simulink library "GUARD_Toolbox"  (R2016a)
settings: Solver=ode45  StartTime=0.0  StopTime=10.0  RelTol=1e-3
undefined symbols (not defined in the file): beta_s, DiscIntNeverNeededParam, k_s, Ts, UW
libraries: vrlib x7, GUARD_Toolbox x3, instrumentlib x1
settings Model: Creator=Marlo  LastModifiedBy=marlo
settings DataIOCC: LimitDataPoints=on
settings DebuggingCC: AllowSymbolicDim=off

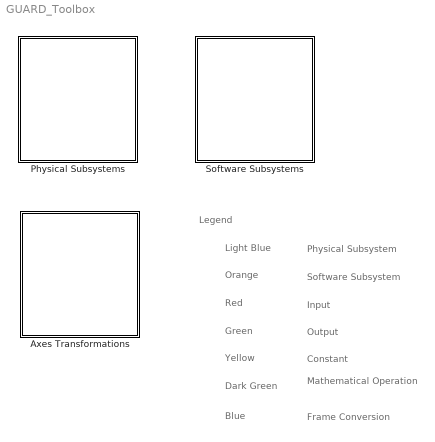
== system GUARD_Toolbox ==
  note: Legend
  note: Physical Subsystem
  note: Light Blue
  note: Red
  note: Input
  note: Green
  note: Output
  note: Yellow
  note: Constant
  note: Dark Green
  note: Mathematical
      | Operation
  note: Software Subsystem
  note: Orange
  note: Blue
  note: Frame Conversion
  Axes Transformations : Subsystem
      mask Display: image(fullfile('Icons','coord_sys.png'));
  Physical Subsystems : Subsystem
      mask Display: image(fullfile('Icons','SS_ISS_low.jpg'));
  Software Subsystems : Subsystem
      mask Display: image(fullfile('Icons','GPAD.png'));

== system GUARD_Toolbox/Axes Transformations ==
  Body to ECI : MATLAB Function  TreatAsAtomicUnit=on  mask(Body to ECI){}
      mask help: Converts a vector in the body frame to an equivalent one in the ECI frame.
  ECI to Body : MATLAB Function  TreatAsAtomicUnit=on  mask(ECI to body){}
      mask help: Converts a vector in the ECI frame to an equivalent one in the body frame.
  From ECEF to ECI : MATLAB Function  TreatAsAtomicUnit=on  mask(ECEF to ECI){}
      mask help: Convert Earth Centered Earth Fixed (ECEF) coordinates to Earth Centered Inertial (ECI) coordinates.
  From ECEF to LLA : MATLAB Function  TreatAsAtomicUnit=on  mask(ECEF to LLA){}
      mask help: Convert Earth Centered Earth Fixed (ECEF) coordinates to Latitude, Longitude, Altitude (LLA) geodetic coordinates.
  From ECI to ECEF : MATLAB Function  TreatAsAtomicUnit=on  mask(ECI to ECEF){}
      mask help: Convert Earth Centered Inertial (ECI) coordinates to Earth Centered Earth Fixed (ECEF) coordinates.
  From ECI to LLA : MATLAB Function  TreatAsAtomicUnit=on  mask(ECI to LLA){}
      mask help: Convert Earth Centered Inertial (ECI) coordinates to Latitude, Longitude, Altitude (LLA) geodetic coordinates.
  From LLA to ECEF : MATLAB Function  TreatAsAtomicUnit=on  mask(LLA to ECEF){}
      mask help: Convert Latitude, Longitude, Altitude (LLA) geodetic coordinates to Earth Centered Earth Fixed (ECEF) coordinates.
  From LVLH to ECI : MATLAB Function  TreatAsAtomicUnit=on  mask(LVLH to ECI){}
      mask help: Convert a vector from the Local Horizontal Local Vertical frame to the Earth Centered Inertial frame.

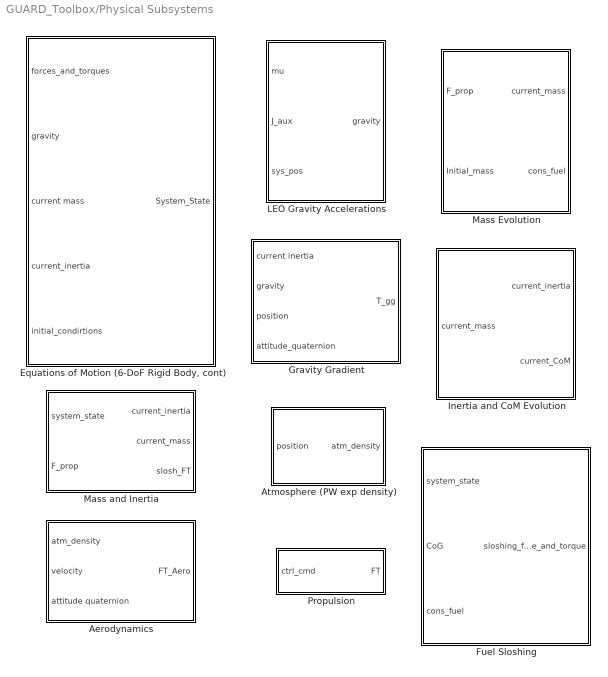
== system GUARD_Toolbox/Physical Subsystems ==
  Aerodynamics : Subsystem  mask(Aerodynamics Model){}
      mask help: Forces and torques enforced on the satellite due to the aerodynamic drag.
  Atmosphere (PW exp density) : Subsystem  mask(Piecewise Atmospheric Model){}
      mask help: U.S. Standard Atmosphere 1976 for 0 [Km], CIRA-72 for 25-500 [Km] and CIRA-72 with exospheric temperature Tinf = 1000 [K] for 500-1000 [Km].
  "Equations of Motion (6-DoF Rigid Body, cont)" : Subsystem  mask(Equatons of Motion){}
      mask help: Non-linear translational and rotational Equations of Motion for a rigid body with six degrees of freedom.
  Fuel Sloshing : Subsystem  mask(Fuel Sloshing){}
      mask help: Compute the disturbance forces and the torques generated by fuel sloshing via a mass-spring-dampener model.
  Gravity Gradient : Subsystem  mask(Gravity Gradient Torque){}
      mask help:
      | Compute the torques acting on the satellite's body due to the gravity gradient. The planet is assumed to be a perfect sphere with radially
      | symmetric mass distribution.
  Inertia and CoM Evolution : Subsystem  mask(Inertia and Center of Mass Evolution){}
      mask help: Interpolated lookup tables to compute the actual inertia matrix and center of mass.
  LEO Gravity Accelerations : MATLAB Function  TreatAsAtomicUnit=on  mask(LEO Gravity Model){}
      mask help: Compute the gravity acceleration vector for a small body in Low Earth Orbit (LEO) taking in account for J2 and J3 zonal harmonics perturbations due to the oblateness of the planet.
  Mass Evolution : Subsystem  mask(Mass Evolution){}
      mask help: Utilizes the forces generated by the propulsion system and the initial mass of the vehicle to compute the actual mass of the satellite and the consumed fuel.
  Mass and Inertia : Subsystem  mask(Preset Mass and Inertia Subsystem){}
      mask help: Mass and Inertia evolution using "Mass Evolution", "Inertia and CoM", and "Fuel Sloshing" blocks.
  Propulsion : Subsystem  mask(Propulson System){}
      mask help: Satellite's propulsion system.

== system GUARD_Toolbox/Software Subsystems ==
  Control Allocation : Subsystem  mask(Controll Allocator){}
      mask help: Allocate actuators.
  GNC : Subsystem  mask(GNC Subsystem){}
      mask help: Guidance Navigation and Control Architecture.
  State Estimation : Subsystem  mask(State Estimation){}
      mask help: Fuse sensors data to estimate the current system's state.
  UE4 OSC_UDP Interface : Subsystem  mask(UE4 OSC_UDP Interface){}
      mask help: Send data to the Unreal Engine 4 using the OSC protocol via UDP network.

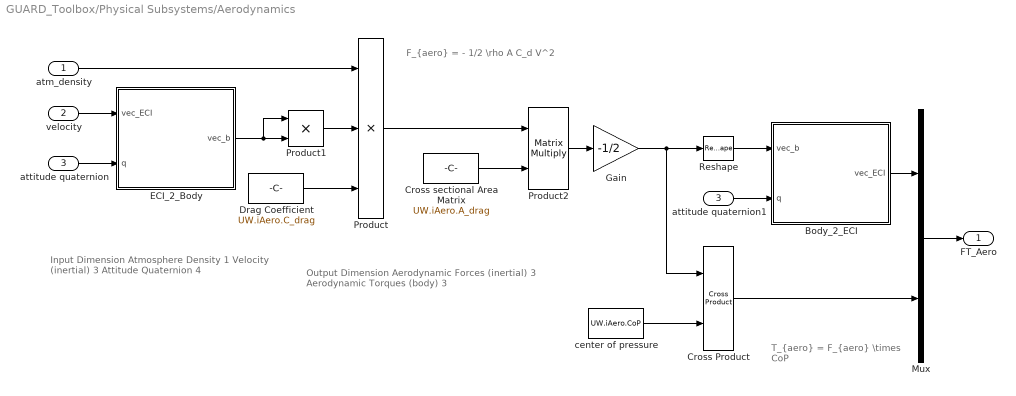
== system GUARD_Toolbox/Physical Subsystems/Aerodynamics ==
  note: F_{aero} = - 1/2 \rho A C_d V^2
  note: Input
      | Dimension
      |
      | Atmosphere Density
      | 1
      |
      | Velocity (inertial)
      | 3
      |
      | Attitude Quaternion
      | 4
  note: Output
      | Dimension
      |
      | Aerodynamic Forces (inertial)
      | 3
      |
      | Aerodynamic Torques (body)
      | 3
  note: T_{aero} = F_{aero} \times CoP
  atm_density : Inport
  velocity : Inport  Port=2
  attitude quaternion : Inport  Port=3
  Body_2_ECI : MATLAB Function  TreatAsAtomicUnit=on
  Cross Product : vrlib/Utilities/Cross Product
  Cross sectional Area Matrix : Constant  Value=UW.iAero.A_drag
  Drag Coefficient : Constant  Value=UW.iAero.C_drag
  ECI_2_Body : MATLAB Function  TreatAsAtomicUnit=on
  Gain : Gain  Gain=-1/2
  Mux : Mux  Inputs=[3 3]
  Product : Product  Inputs=***  SaturateOnIntegerOverflow=on  RndMeth=Zero  InputSameDT=on  OutDataTypeStr=Inherit: Same as first input
  Product1 : Product  Inputs=**  SaturateOnIntegerOverflow=on  RndMeth=Zero  InputSameDT=on  OutDataTypeStr=Inherit: Same as first input
  Product2 : Product  Inputs=**  Multiplication=Matrix(*)  SaturateOnIntegerOverflow=on  RndMeth=Zero  InputSameDT=on  OutDataTypeStr=Inherit: Same as first input
  Reshape : Reshape  OutputDimensionality=Column vector (2-D)
  attitude quaternion1 : InportShadow  Port=3
  center of pressure : Constant  Value=UW.iAero.CoP
  FT_Aero : Outport
  wires:
  Drag Coefficient/1 -> Product/3
  atm_density/1 -> Product/1
  Product1/1 -> Product/2
  Product/1 -> Product2/1
  Cross sectional Area Matrix/1 -> Product2/2
  Gain/1 -> Reshape/1, Cross Product/1
  Product2/1 -> Gain/1
  Cross Product/1 -> Mux/2
  velocity/1 -> ECI_2_Body/1(vec_ECI)
  attitude quaternion/1 -> ECI_2_Body/2(q)
  ECI_2_Body/1(vec_b) -> Product1/2, Product1/1
  center of pressure/1 -> Cross Product/2
  attitude quaternion1/1 -> Body_2_ECI/2(q)
  Body_2_ECI/1(vec_ECI) -> Mux/1
  Mux/1 -> FT_Aero/1
  Reshape/1 -> Body_2_ECI/1(vec_b)

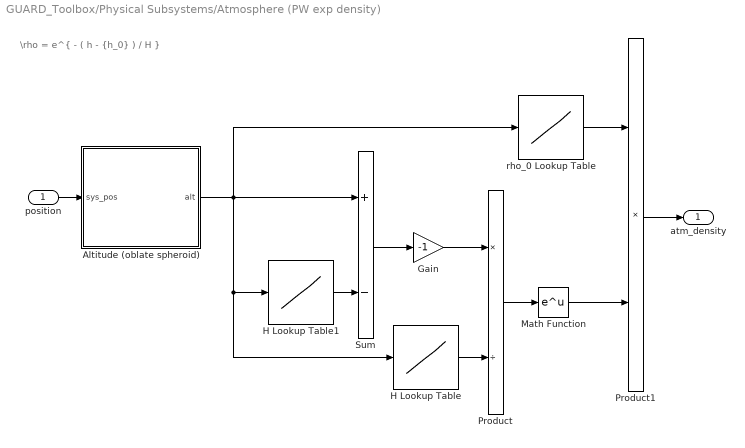
== system GUARD_Toolbox/Physical Subsystems/Atmosphere (PW exp density) ==
  note: \rho = e^{ - ( h - {h_0} ) / H }
  position : Inport
  Altitude (oblate spheroid) : MATLAB Function  TreatAsAtomicUnit=on
  Gain : Gain  Gain=-1
  H Lookup Table : Lookup_n-D  NumberOfTableDimensions=1  BreakpointsForDimension1=UW.iPWatm.h_idx  Table=UW.iPWatm.H  InternalRulePriority=Speed  RndMeth=Simplest  InputSameDT=on
  H Lookup Table1 : Lookup_n-D  NumberOfTableDimensions=1  BreakpointsForDimension1=UW.iPWatm.h_idx  Table=UW.iPWatm.h_idx  InternalRulePriority=Speed  RndMeth=Simplest  InputSameDT=on
  Math Function : Math  SaturateOnIntegerOverflow=on
  Product : Product  Inputs=*/  SaturateOnIntegerOverflow=on  RndMeth=Zero  InputSameDT=on  OutDataTypeStr=Inherit: Same as first input
  Product1 : Product  Inputs=**  SaturateOnIntegerOverflow=on  RndMeth=Zero  InputSameDT=on  OutDataTypeStr=Inherit: Same as first input
  Sum : Sum  Inputs=+-
  rho_0 Lookup Table : Lookup_n-D  NumberOfTableDimensions=1  BreakpointsForDimension1=UW.iPWatm.h_idx  Table=UW.iPWatm.rho_0  InternalRulePriority=Speed  RndMeth=Simplest  InputSameDT=on
  atm_density : Outport
  wires:
  Product1/1 -> atm_density/1
  position/1 -> Altitude (oblate spheroid)/1(sys_pos)
  Altitude (oblate spheroid)/1(alt) -> Sum/1, rho_0 Lookup Table/1, H Lookup Table/1, H Lookup Table1/1
  Sum/1 -> Gain/1
  Gain/1 -> Product/1
  H Lookup Table/1 -> Product/2
  Product/1 -> Math Function/1
  Math Function/1 -> Product1/2
  rho_0 Lookup Table/1 -> Product1/1
  H Lookup Table1/1 -> Sum/2

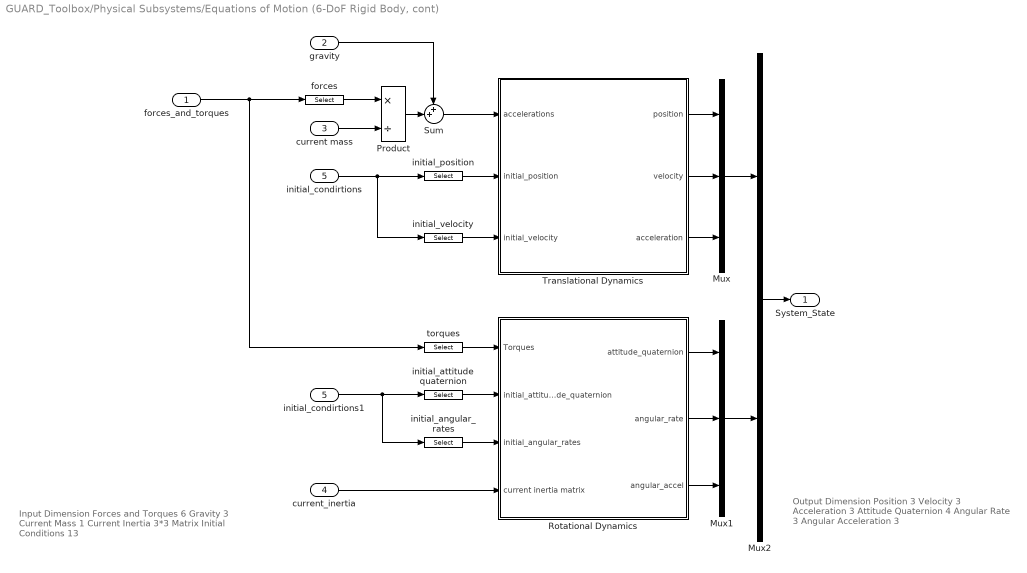
== system GUARD_Toolbox/Physical Subsystems/Equations of Motion (6-DoF Rigid Body, cont) ==
  note: Output
      | Dimension
      |
      | Position
      | 3
      |
      | Velocity
      | 3
      |
      | Acceleration
      | 3
      |
      | Attitude Quaternion
      | 4
      |
      | Angular Rate
      | 3
      |
      | Angular Acceleration
      | 3
  note: Input
      | Dimension
      |
      | Forces and Torques
      | 6
      |
      | Gravity
      | 3
      |
      | Current Mass
      | 1
      |
      | Current Inertia
      | 3*3 Matrix
      |
      | Initial Conditions
      | 13
  forces_and_torques : Inport
  gravity : Inport  Port=2
  current mass : Inport  Port=3  PortDimensions=1
  current_inertia : Inport  Port=4
  initial_condirtions : Inport  Port=5
  Mux : Mux  Inputs=[3 3 3]
  Mux1 : Mux  Inputs=[4 3 3]
  Mux2 : Mux  Inputs=[9 10]
  Product : Product  Inputs=*/  SaturateOnIntegerOverflow=on  RndMeth=Zero  InputSameDT=on  OutDataTypeStr=Inherit: Same as first input
  Rotational Dynamics : Subsystem
  Sum : Sum  Inputs=++|
  Translational Dynamics : Subsystem
  forces : Selector  InputPortWidth=6  IndexOptions=Index vector (dialog)  Indices=[1 2 3]  OutputSizes=1
  initial_angular_rates : Selector  InputPortWidth=13  IndexOptions=Index vector (dialog)  Indices=[11 12 13]  OutputSizes=1
  initial_attitude quaternion : Selector  InputPortWidth=13  IndexOptions=Index vector (dialog)  Indices=[7 8 9 10]  OutputSizes=1
  initial_condirtions1 : InportShadow  Port=5
  initial_position : Selector  InputPortWidth=13  IndexOptions=Index vector (dialog)  Indices=[1 2 3]  OutputSizes=1
  initial_velocity : Selector  InputPortWidth=13  IndexOptions=Index vector (dialog)  Indices=[4 5 6]  OutputSizes=1
  torques : Selector  InputPortWidth=6  IndexOptions=Index vector (dialog)  Indices=[4 5 6]  OutputSizes=1
  System_State : Outport
  wires:
  Mux1/1 -> Mux2/2
  Mux/1 -> Mux2/1
  Rotational Dynamics/1(attitude_quaternion) -> Mux1/1
  Rotational Dynamics/2(angular_rate) -> Mux1/2
  Rotational Dynamics/3(angular_accel) -> Mux1/3
  Translational Dynamics/1(position) -> Mux/1
  Translational Dynamics/2(velocity) -> Mux/2
  Translational Dynamics/3(acceleration) -> Mux/3
  Mux2/1 -> System_State/1
  initial_condirtions1/1 -> initial_attitude quaternion/1, initial_angular_rates/1
  initial_condirtions/1 -> initial_position/1, initial_velocity/1
  initial_attitude quaternion/1 -> Rotational Dynamics/2(initial_attitude_quaternion)
  initial_angular_rates/1 -> Rotational Dynamics/3(initial_angular_rates)
  initial_velocity/1 -> Translational Dynamics/3(initial_velocity)
  initial_position/1 -> Translational Dynamics/2(initial_position)
  current_inertia/1 -> Rotational Dynamics/4(current inertia matrix)
  torques/1 -> Rotational Dynamics/1(Torques)
  forces_and_torques/1 -> torques/1, forces/1
  gravity/1 -> Sum/1
  Sum/1 -> Translational Dynamics/1(accelerations)
  forces/1 -> Product/1
  current mass/1 -> Product/2
  Product/1 -> Sum/2

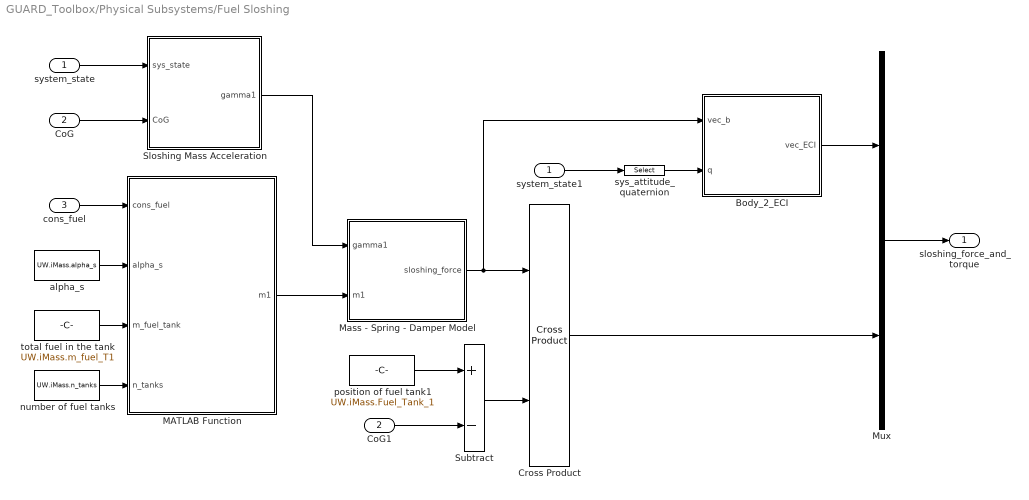
== system GUARD_Toolbox/Physical Subsystems/Fuel Sloshing ==
  system_state : Inport
  CoG : Inport  Port=2
  cons_fuel : Inport  Port=3
  Body_2_ECI : MATLAB Function  TreatAsAtomicUnit=on
  CoG1 : InportShadow  Port=2
  Cross Product : vrlib/Utilities/Cross Product
  MATLAB Function : MATLAB Function  TreatAsAtomicUnit=on
  Mass - Spring - Damper Model : Subsystem
  Mux : Mux  Inputs=[3 3]
  Sloshing Mass Acceleration : Subsystem
  Subtract : Sum  Inputs=+-
  alpha_s : Constant  Value=UW.iMass.alpha_s
  number of fuel tanks : Constant  Value=UW.iMass.n_tanks
  position of fuel tank1 : Constant  Value=UW.iMass.Fuel_Tank_1
  sys_attitude_quaternion : Selector  InputPortWidth=19  IndexOptions=Index vector (dialog)  Indices=[10 11 12 13]  OutputSizes=1
  system_state1 : InportShadow
  total fuel in the tank : Constant  Value=UW.iMass.m_fuel_T1
  sloshing_force_and_torque : Outport
  wires:
  system_state1/1 -> sys_attitude_quaternion/1
  sys_attitude_quaternion/1 -> Body_2_ECI/2(q)
  Sloshing Mass Acceleration/1(gamma1) -> Mass - Spring - Damper Model/1(gamma1)
  CoG1/1 -> Subtract/2
  position of fuel tank1/1 -> Subtract/1
  system_state/1 -> Sloshing Mass Acceleration/1(sys_state)
  CoG/1 -> Sloshing Mass Acceleration/2(CoG)
  Mux/1 -> sloshing_force_and_torque/1
  Body_2_ECI/1(vec_ECI) -> Mux/1
  Cross Product/1 -> Mux/2
  Subtract/1 -> Cross Product/2
  Mass - Spring - Damper Model/1(sloshing_force) -> Body_2_ECI/1(vec_b), Cross Product/1
  number of fuel tanks/1 -> MATLAB Function/4(n_tanks)
  cons_fuel/1 -> MATLAB Function/1(cons_fuel)
  MATLAB Function/1(m1) -> Mass - Spring - Damper Model/2(m1)
  total fuel in the tank/1 -> MATLAB Function/3(m_fuel_tank)
  alpha_s/1 -> MATLAB Function/2(alpha_s)

== system GUARD_Toolbox/Physical Subsystems/Gravity Gradient ==
  note: T_{gg} = 3 \mu / r^3 \bf{o_3} \times I o_3
  note: Output
      | Dimension
      |
      | Gravity Gradient Torque (body)
      | 3
  note: Input
      | Dimension
      |
      | Current Inertia
      | 3*3
      |
      | Position (inertial)
      | 3
      |
      | Attitude Quaternion
      | 4
  current inertia : Inport
  gravity : Inport  Port=2
  position : Inport  Port=3
  attitude_quaternion : Inport  Port=4
  ECI to Body : MATLAB Function  TreatAsAtomicUnit=on  mask(ECI to body){}
      mask help: Converts a vector in the ECI frame to an equivalent one in the body frame.
  Gravity Gradient Torque : MATLAB Function  TreatAsAtomicUnit=on
  gravitaitonal parameter : Constant  Value=UW.iPlanet.mu
  T_gg : Outport
  wires:
  current inertia/1 -> Gravity Gradient Torque/4(current_inertia)
  Gravity Gradient Torque/1(ggt) -> T_gg/1
  gravity/1 -> ECI to Body/1(vec_ECI)
  attitude_quaternion/1 -> ECI to Body/2(q)
  ECI to Body/1(vec_b) -> Gravity Gradient Torque/1(gravity_body)
  position/1 -> Gravity Gradient Torque/2(sys_pos)
  gravitaitonal parameter/1 -> Gravity Gradient Torque/3(mu)

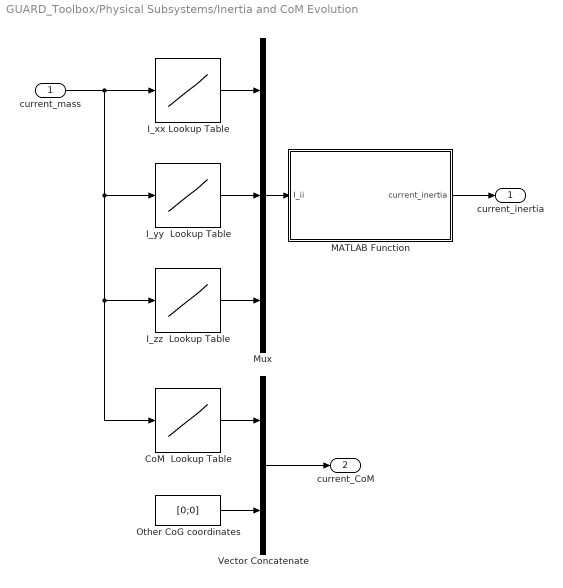
== system GUARD_Toolbox/Physical Subsystems/Inertia and CoM Evolution ==
  current_mass : Inport
  CoM  Lookup Table : Lookup_n-D  NumberOfTableDimensions=1  BreakpointsForDimension1=UW.iMass.m_idx  Table=UW.iMass.GoG_m  InternalRulePriority=Speed  RndMeth=Simplest  InputSameDT=on
  I_xx Lookup Table : Lookup_n-D  NumberOfTableDimensions=1  BreakpointsForDimension1=UW.iMass.m_idx  Table=UW.iMass.I_xx_m  InternalRulePriority=Speed  RndMeth=Simplest  InputSameDT=on
  I_yy  Lookup Table : Lookup_n-D  NumberOfTableDimensions=1  BreakpointsForDimension1=UW.iMass.m_idx  Table=UW.iMass.I_yy_m  InternalRulePriority=Speed  RndMeth=Simplest  InputSameDT=on
  I_zz  Lookup Table : Lookup_n-D  NumberOfTableDimensions=1  BreakpointsForDimension1=UW.iMass.m_idx  Table=UW.iMass.I_zz_m  InternalRulePriority=Speed  RndMeth=Simplest  InputSameDT=on
  MATLAB Function : MATLAB Function  TreatAsAtomicUnit=on
  Mux : Mux  Inputs=3
  Other CoG coordinates : Constant  Value=[0;0]
  Vector Concatenate : Concatenate
  current_inertia : Outport
  current_CoM : Outport  Port=2
  wires:
  Other CoG coordinates/1 -> Vector Concatenate/2
  Vector Concatenate/1 -> current_CoM/1
  CoM  Lookup Table/1 -> Vector Concatenate/1
  MATLAB Function/1(current_inertia) -> current_inertia/1
  I_yy  Lookup Table/1 -> Mux/2
  I_xx Lookup Table/1 -> Mux/1
  I_zz  Lookup Table/1 -> Mux/3
  current_mass/1 -> I_xx Lookup Table/1, I_zz  Lookup Table/1, CoM  Lookup Table/1, I_yy  Lookup Table/1
  Mux/1 -> MATLAB Function/1(I_ii)

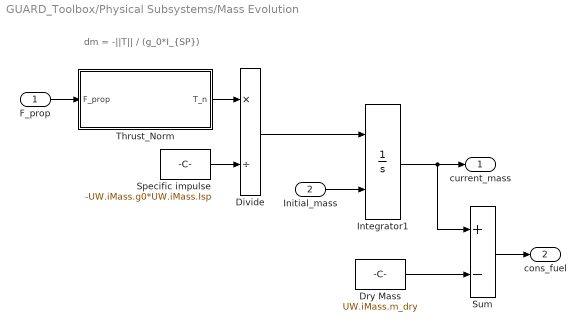
== system GUARD_Toolbox/Physical Subsystems/Mass Evolution ==
  note: dm = -||T|| / (g_0*I_{SP})
  F_prop : Inport
  Initial_mass : Inport  Port=2
  Divide : Product  Inputs=*/
  Dry Mass : Constant  Value=UW.iMass.m_dry
  Integrator1 : Integrator  InitialConditionSource=external
  Specific impulse : Constant  Value=-UW.iMass.g0*UW.iMass.Isp
  Sum : Sum  Inputs=+-
  Thrust_Norm : MATLAB Function  TreatAsAtomicUnit=on
  current_mass : Outport
  cons_fuel : Outport  Port=2
  wires:
  Dry Mass/1 -> Sum/2
  Sum/1 -> cons_fuel/1
  Integrator1/1 -> current_mass/1, Sum/1
  Initial_mass/1 -> Integrator1/2
  F_prop/1 -> Thrust_Norm/1(F_prop)
  Thrust_Norm/1(T_n) -> Divide/1
  Specific impulse/1 -> Divide/2
  Divide/1 -> Integrator1/1

== system GUARD_Toolbox/Physical Subsystems/Mass and Inertia ==
  note: Input
      | Dimension
      |
      | Propulsion system Forces
      | 3
      |
      | system state
      | 19
  note: Output
      | Dimension
      |
      | Sloshing Forces and Torques
      | 3
      |
      | Current Mass
      | 1
      |
      | Current inertia Matrix
      | 3*3
  system_state : Inport
  F_prop : Inport  Port=2
  Fuel Sloshing : GUARD_Toolbox/Physical Subsystems/Fuel Sloshing  Commented=on
  Inertia and CoM Evolution : GUARD_Toolbox/Physical Subsystems/Inertia and CoM Evolution
  Mass Evolution : GUARD_Toolbox/Physical Subsystems/Mass Evolution
  initial_mass : Constant  Value=UW.iMass.m_wet
  current_inertia : Outport
  current_mass : Outport  Port=2
  slosh_FT : Outport  Port=3
  wires:
  Mass Evolution/1 -> Inertia and CoM Evolution/1, current_mass/1
  F_prop/1 -> Mass Evolution/1
  initial_mass/1 -> Mass Evolution/2
  Inertia and CoM Evolution/1 -> current_inertia/1
  Fuel Sloshing/1 -> slosh_FT/1
  system_state/1 -> Fuel Sloshing/1
  Mass Evolution/2 -> Fuel Sloshing/3
  Inertia and CoM Evolution/2 -> Fuel Sloshing/2

== system GUARD_Toolbox/Physical Subsystems/Propulsion ==
  note: Output
      | Dimension
      |
      | Attained Forces and Torques
      | 6
  ctrl_cmd : Inport
  FT : Outport
  wires:
  ctrl_cmd/1 -> FT/1

== system GUARD_Toolbox/Software Subsystems/Control Allocation ==
  GNC_FT : Inport
  ctr_cmd : Outport
  wires:
  GNC_FT/1 -> ctr_cmd/1

== system GUARD_Toolbox/Software Subsystems/GNC ==
  est_state : Inport
  Feedback Controller : Subsystem
  Guidance : Subsystem
  GNC_FT : Outport
  wires:
  Feedback Controller/1(Out1) -> GNC_FT/1
  Guidance/1(Out1) -> Feedback Controller/1(guidance_cmd)
  est_state/1 -> Guidance/1(In1), Feedback Controller/2(est_state)

== system GUARD_Toolbox/Software Subsystems/State Estimation ==
  note: Output
      | Dimension
      |
      | Estimated System State
      | ?
  note: Input
      | Dimension
      |
      | Sensed System State
      | ?
  sens_state : Inport
  est_state : Outport
  wires:
  sens_state/1 -> est_state/1

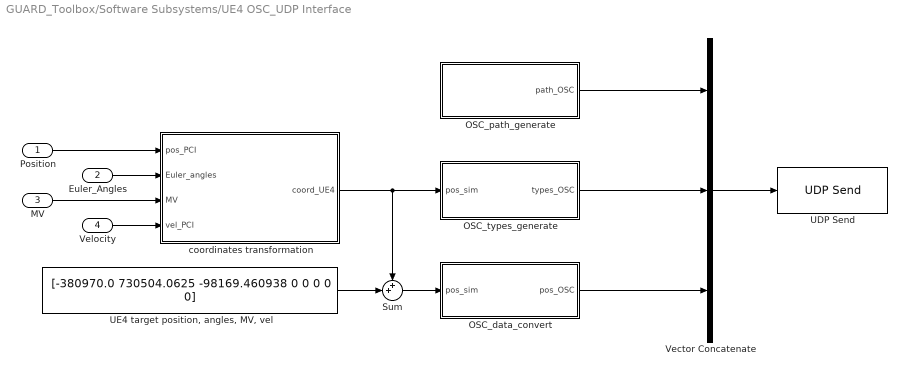
== system GUARD_Toolbox/Software Subsystems/UE4 OSC_UDP Interface ==
  Position : Inport
  Euler_Angles : Inport  Port=2
  MV : Inport  Port=3
  Velocity : Inport  Port=4
  OSC_data_convert : MATLAB Function  TreatAsAtomicUnit=on
  OSC_path_generate : MATLAB Function  TreatAsAtomicUnit=on
  OSC_types_generate : MATLAB Function  TreatAsAtomicUnit=on
  Sum : Sum  Inputs=++|
  UDP Send : instrumentlib/UDP Send  Host=127.0.0.1  Port=8000  LocalPort=-1  EnableBlockingMode=on  ByteOrder=BigEndian
  "UE4 target position, angles, MV, vel" : Constant  Value=[-380970.0 730504.0625 -98169.460938 0 0 0 0 0]  VectorParams1D=off
  Vector Concatenate : Concatenate  NumInputs=3
  coordinates transformation : MATLAB Function  TreatAsAtomicUnit=on
  wires:
  Velocity/1 -> coordinates transformation/4(vel_PCI)
  MV/1 -> coordinates transformation/3(MV)
  Vector Concatenate/1 -> UDP Send/1
  Euler_Angles/1 -> coordinates transformation/2(Euler_angles)
  Position/1 -> coordinates transformation/1(pos_PCI)
  coordinates transformation/1(coord_UE4) -> OSC_types_generate/1(pos_sim), Sum/1
  Sum/1 -> OSC_data_convert/1(pos_sim)
  "UE4 target position, angles, MV, vel"/1 -> Sum/2
  OSC_data_convert/1(pos_OSC) -> Vector Concatenate/3
  OSC_types_generate/1(types_OSC) -> Vector Concatenate/2
  OSC_path_generate/1(path_OSC) -> Vector Concatenate/1

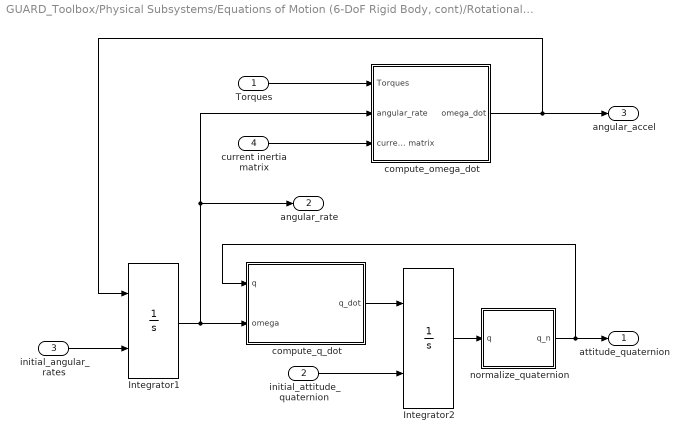
== system GUARD_Toolbox/Physical Subsystems/Equations of Motion (6-DoF Rigid Body, cont)/Rotational Dynamics ==
  Torques : Inport
  initial_attitude_quaternion : Inport  Port=2
  initial_angular_rates : Inport  Port=3
  current inertia matrix : Inport  Port=4
  Integrator1 : Integrator  InitialConditionSource=external
  Integrator2 : Integrator  InitialConditionSource=external
  compute_omega_dot : Subsystem
  compute_q_dot : MATLAB Function  TreatAsAtomicUnit=on
  normalize_quaternion : MATLAB Function  TreatAsAtomicUnit=on
  attitude_quaternion : Outport
  angular_rate : Outport  Port=2
  angular_accel : Outport  Port=3
  wires:
  Torques/1 -> compute_omega_dot/1(Torques)
  normalize_quaternion/1(q_n) -> attitude_quaternion/1, compute_q_dot/1(q)
  Integrator2/1 -> normalize_quaternion/1(q)
  compute_omega_dot/1(omega_dot) -> Integrator1/1, angular_accel/1
  initial_attitude_quaternion/1 -> Integrator2/2
  compute_q_dot/1(q_dot) -> Integrator2/1
  initial_angular_rates/1 -> Integrator1/2
  current inertia matrix/1 -> compute_omega_dot/3(current inertia matrix)
  Integrator1/1 -> compute_q_dot/2(omega), angular_rate/1, compute_omega_dot/2(angular_rate)

== system GUARD_Toolbox/Physical Subsystems/Equations of Motion (6-DoF Rigid Body, cont)/Translational Dynamics ==
  accelerations : Inport
  initial_position : Inport  Port=2
  initial_velocity : Inport  Port=3
  Integrator : Integrator  InitialConditionSource=external
  Integrator1 : Integrator  InitialConditionSource=external
  position : Outport
  velocity : Outport  Port=2
  acceleration : Outport  Port=3
  wires:
  initial_position/1 -> Integrator1/2
  initial_velocity/1 -> Integrator/2
  Integrator1/1 -> position/1
  accelerations/1 -> Integrator/1, acceleration/1
  Integrator/1 -> Integrator1/1, velocity/1

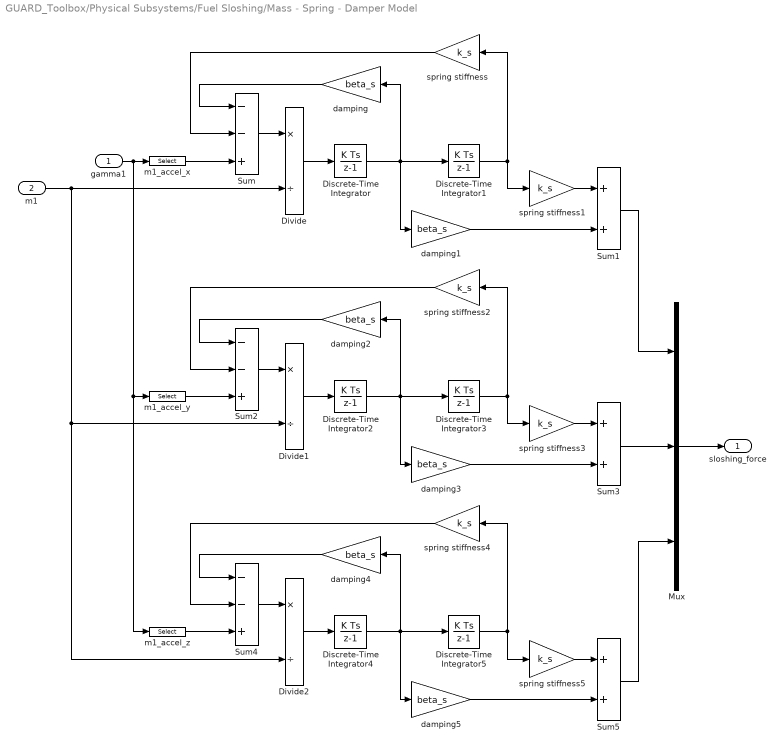
== system GUARD_Toolbox/Physical Subsystems/Fuel Sloshing/Mass - Spring - Damper Model ==
  gamma1 : Inport
  m1 : Inport  Port=2
  Discrete-Time Integrator{,1..5} (6 alike) : DiscreteIntegrator  InitialConditionSetting=State (most efficient)  SampleTime=Ts  ICPrevOutput=DiscIntNeverNeededParam  ICPrevScaledInput=DiscIntNeverNeededParam
  Divide : Product  Inputs=*/
  Divide1 : Product  Inputs=*/
  Divide2 : Product  Inputs=*/
  Mux : Mux  Inputs=3
  Sum : Sum  Inputs=--+
  Sum1 : Sum
  Sum2 : Sum  Inputs=--+
  Sum3 : Sum
  Sum4 : Sum  Inputs=--+
  Sum5 : Sum
  damping{,1..5} (6 alike) : Gain  Gain=beta_s
  m1_accel_x : Selector  InputPortWidth=3  IndexOptions=Index vector (dialog)  Indices=[1]  OutputSizes=1
  m1_accel_y : Selector  InputPortWidth=3  IndexOptions=Index vector (dialog)  Indices=[2]  OutputSizes=1
  m1_accel_z : Selector  InputPortWidth=3  IndexOptions=Index vector (dialog)  Indices=[3]  OutputSizes=1
  spring stiffness{,1..5} (6 alike) : Gain  Gain=k_s
  sloshing_force : Outport
  wires:
  Sum1/1 -> Mux/1
  Mux/1 -> sloshing_force/1
  m1_accel_x/1 -> Sum/3
  damping5/1 -> Sum5/2
  Discrete-Time Integrator5/1 -> spring stiffness4/1, spring stiffness5/1
  Discrete-Time Integrator4/1 -> Discrete-Time Integrator5/1, damping4/1, damping5/1
  Divide2/1 -> Discrete-Time Integrator4/1
  Sum4/1 -> Divide2/1
  spring stiffness4/1 -> Sum4/2
  damping4/1 -> Sum4/1
  spring stiffness5/1 -> Sum5/1
  Sum5/1 -> Mux/3
  m1_accel_z/1 -> Sum4/3
  m1/1 -> Divide/2, Divide1/2, Divide2/2
  damping3/1 -> Sum3/2
  Discrete-Time Integrator3/1 -> spring stiffness3/1, spring stiffness2/1
  Discrete-Time Integrator2/1 -> damping3/1, damping2/1, Discrete-Time Integrator3/1
  Divide1/1 -> Discrete-Time Integrator2/1
  Sum2/1 -> Divide1/1
  spring stiffness2/1 -> Sum2/2
  damping2/1 -> Sum2/1
  spring stiffness3/1 -> Sum3/1
  Sum3/1 -> Mux/2
  m1_accel_y/1 -> Sum2/3
  damping1/1 -> Sum1/2
  Discrete-Time Integrator1/1 -> spring stiffness1/1, spring stiffness/1
  Discrete-Time Integrator/1 -> damping1/1, damping/1, Discrete-Time Integrator1/1
  Divide/1 -> Discrete-Time Integrator/1
  Sum/1 -> Divide/1
  spring stiffness/1 -> Sum/2
  damping/1 -> Sum/1
  spring stiffness1/1 -> Sum1/1
  gamma1/1 -> m1_accel_x/1, m1_accel_y/1, m1_accel_z/1

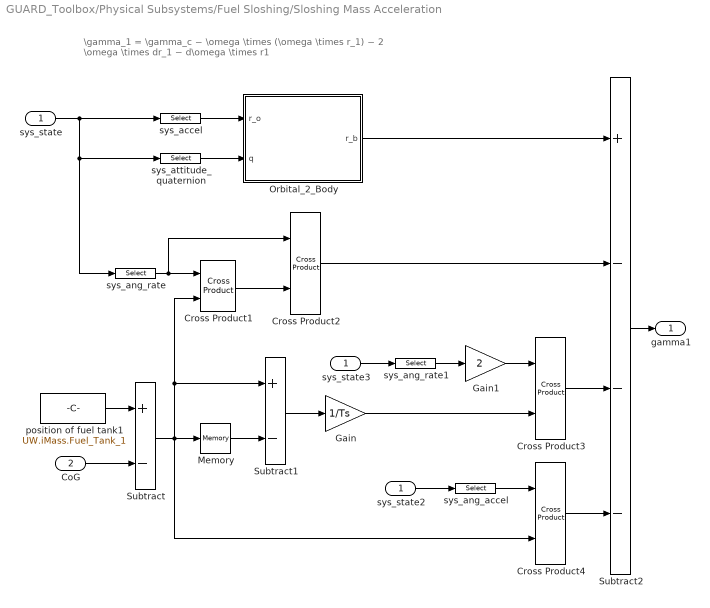
== system GUARD_Toolbox/Physical Subsystems/Fuel Sloshing/Sloshing Mass Acceleration ==
  note: \gamma_1 = \gamma_c − \omega \times (\omega \times r_1) − 2 \omega \times dr_1 − d\omega \times r1
  sys_state : Inport
  CoG : Inport  Port=2
  Cross Product{1..4} (4 alike) : vrlib/Utilities/Cross Product
  Gain : Gain  Gain=1/Ts
  Gain1 : Gain  Gain=2
  Memory : Memory  X0=UW.iMass.Fuel_Tank_1
  Orbital_2_Body : MATLAB Function  TreatAsAtomicUnit=on
  Subtract : Sum  Inputs=+-
  Subtract1 : Sum  Inputs=+-
  Subtract2 : Sum  Inputs=+---
  position of fuel tank1 : Constant  Value=UW.iMass.Fuel_Tank_1
  sys_accel : Selector  InputPortWidth=19  IndexOptions=Index vector (dialog)  Indices=[7 8 9]  OutputSizes=1
  sys_ang_accel : Selector  InputPortWidth=19  IndexOptions=Index vector (dialog)  Indices=[17 18 19]  OutputSizes=1
  sys_ang_rate : Selector  InputPortWidth=19  IndexOptions=Index vector (dialog)  Indices=[14 15 16]  OutputSizes=1
  sys_ang_rate1 : Selector  InputPortWidth=19  IndexOptions=Index vector (dialog)  Indices=[14 15 16]  OutputSizes=1
  sys_attitude_quaternion : Selector  InputPortWidth=19  IndexOptions=Index vector (dialog)  Indices=[10 11 12 13]  OutputSizes=1
  sys_state2 : InportShadow
  sys_state3 : InportShadow
  gamma1 : Outport
  wires:
  Cross Product3/1 -> Subtract2/3
  Cross Product4/1 -> Subtract2/4
  Gain1/1 -> Cross Product3/1
  Subtract1/1 -> Gain/1
  sys_state2/1 -> sys_ang_accel/1
  sys_state3/1 -> sys_ang_rate1/1
  sys_ang_rate1/1 -> Gain1/1
  sys_ang_accel/1 -> Cross Product4/1
  Gain/1 -> Cross Product3/2
  Subtract2/1 -> gamma1/1
  sys_state/1 -> sys_accel/1, sys_ang_rate/1, sys_attitude_quaternion/1
  sys_accel/1 -> Orbital_2_Body/1(r_o)
  sys_attitude_quaternion/1 -> Orbital_2_Body/2(q)
  Subtract/1 -> Memory/1, Subtract1/1, Cross Product1/2, Cross Product4/2
  Cross Product2/1 -> Subtract2/2
  Orbital_2_Body/1(r_b) -> Subtract2/1
  sys_ang_rate/1 -> Cross Product1/1, Cross Product2/1
  CoG/1 -> Subtract/2
  position of fuel tank1/1 -> Subtract/1
  Cross Product1/1 -> Cross Product2/2
  Memory/1 -> Subtract1/2

== system GUARD_Toolbox/Software Subsystems/GNC/Feedback Controller ==
  guidance_cmd : Inport
  est_state : Inport  Port=2
  Out1 : Outport

== system GUARD_Toolbox/Software Subsystems/GNC/Guidance ==
  In1 : Inport
  Out1 : Outport

== system GUARD_Toolbox/Physical Subsystems/Equations of Motion (6-DoF Rigid Body, cont)/Rotational Dynamics/compute_omega_dot ==
  note: 3*3 I matrix
  note: I omega
  note: omega
  Torques : Inport
  angular_rate : Inport  Port=2
  current inertia matrix : Inport  Port=3
  -inv(Inertia)*omega x Inertia*omega + T : Product  Multiplication=Matrix(*)  SaturateOnIntegerOverflow=on  RndMeth=Zero  InputSameDT=on  OutDataTypeStr=Inherit: Same as first input
  Inertia*omega : Product  Multiplication=Matrix(*)  SaturateOnIntegerOverflow=on  RndMeth=Zero  InputSameDT=on  OutDataTypeStr=Inherit: Same as first input
  Sum : Sum  Inputs=+-
  cross_product : vrlib/Utilities/Cross Product
  inv(Inertia) : Product  Inputs=/  Multiplication=Matrix(*)  SaturateOnIntegerOverflow=on  RndMeth=Zero  InputSameDT=on  OutDataTypeStr=Inherit: Same as first input
  omega_dot : Outport
  wires:
  inv(Inertia)/1 -> -inv(Inertia)*omega x Inertia*omega + T/1
  current inertia matrix/1 -> Inertia*omega/1, inv(Inertia)/1
  cross_product/1 -> Sum/2
  -inv(Inertia)*omega x Inertia*omega + T/1 -> omega_dot/1
  Sum/1 -> -inv(Inertia)*omega x Inertia*omega + T/2
  Torques/1 -> Sum/1
  Inertia*omega/1 -> cross_product/2
  angular_rate/1 -> cross_product/1, Inertia*omega/2

== matlab function GUARD_Toolbox/Physical Subsystems/LEO Gravity Accelerations ==
  data: mu input; J_aux input; gravity output; sys_pos input
function gravity = gravity_acc(mu,J_aux,sys_pos)
%#codegen

% ECI frame
X = sys_pos(1);
Y = sys_pos(2);
Z = sys_pos(3);

% offline zonal harmonics terms
J2_aux = J_aux(1);
J3_aux = J_aux(2);
% Spacecraft distance from the planet's center
r = sqrt(X^2 + Y^2 + Z^2);

% spherical Earth;
kep_acc = mu/r^3;

% J2 perturbation
a = J2_aux/(r^7);
b = 5*Z^2;
J2_pert_XY = (b - r^2)*[X;Y];
J2_pert_Z = (b - 3*r^2)*Z;
J2_pert = a*[J2_pert_XY;J2_pert_Z];

% J3 perturbation

c = J3_aux/r^9;

J3_pert_XY = 5*Z*(7*Z^2 - 3*r^2)*[X;Y];
J3_pert_Z = 35*Z^4 - 30*Z^2*r^2 + 3*r^4;
J3_pert = c*[J3_pert_XY;J3_pert_Z];

gravity=-kep_acc*sys_pos + J2_pert + J3_pert;

% J2
%         2          2    2
% 3 J2 r_E  X mu (5 Z  - r )
% -------------------------
%              7
%           2 r
% 
%         2          2    2
% 3 J2 r_E  Y mu (5 Z  - r )
% -------------------------
%              7
%           2 r
% 
%         2          2      2
% 3 J2 r_E  Z mu (5 Z  - 3 r )
% ---------------------------
%               7
%            2 r

% J3
%       3            2       2
% 5 J3 R  X Z mu (7 Z  - 3 rs )
% -----------------------------
%                 9
%             2 rs
% 
%       3            2       2
% 5 J3 R  Y Z mu (7 Z  - 3 rs )
% -----------------------------
%                 9
%             2 rs
% 
%     3         4       2   2       4
% J3 R  mu (35 Z  - 30 Z  rs  + 3 rs )
% ------------------------------------
%                     9
%                 2 rs

== matlab function GUARD_Toolbox/Physical Subsystems/Gravity Gradient/ECI to Body ==
  settings: sampleTime=Tsc
  data: vec_ECI input; q input; vec_b output
function  vec_b = ECI_to_body(vec_ECI,q)
%#codegen

% Rotate a vector from the orbital frame to the body frame 
% C_bo = Quaternion rotation matrix
% vec_b = Body frame vector
% vec_ECI = Earth Fixed Inertial frame vector
% q   = Attitude quaternion
q1=q(1);
q2=q(2);
q3=q(3);
q4=q(4);

C_b_ECI = [ -2*q2^2 - 2*q3^2 + 1,  2*q1*q2 + 2*q3*q4,    2*q1*q3 - 2*q2*q4;
          2*q1*q2 - 2*q3*q4,   -2*q1^2 - 2*q3^2 + 1,  2*q1*q4 + 2*q2*q3;
          2*q1*q3 + 2*q2*q4,    2*q2*q3 - 2*q1*q4,   -2*q1^2 - 2*q2^2 + 1];
 
vec_b = C_b_ECI*vec_ECI;

== matlab function GUARD_Toolbox/Physical Subsystems/Mass Evolution/Thrust_Norm ==
  data: F_prop input; T_n output
function T_n = T_norm(F_prop)
%#codegen

T_n=sqrt(F_prop(1)^2 + F_prop(2)^2 + F_prop(3)^2);

== matlab function GUARD_Toolbox/Physical Subsystems/Aerodynamics/Body_2_ECI ==
  settings: sampleTime=Tsc
  data: vec_b input; q input; vec_ECI output
function  vec_ECI = body_to_ECI(vec_b,q)
%#codegen

% Rotate a vector from the orbital frame to the body frame 
% C_bo = Quaternion rotation matrix
% vec_b = Body frame vector
% vec_ECI = Earth Fixed Inertial frame vector
% q   = Attitude quaternion
q1=q(1);
q2=q(2);
q3=q(3);
q4=q(4);

C_b_ECI = [ -2*q2^2 - 2*q3^2 + 1,  2*q1*q2 + 2*q3*q4,    2*q1*q3 - 2*q2*q4;
          2*q1*q2 - 2*q3*q4,   -2*q1^2 - 2*q3^2 + 1,  2*q1*q4 + 2*q2*q3;
          2*q1*q3 + 2*q2*q4,    2*q2*q3 - 2*q1*q4,   -2*q1^2 - 2*q2^2 + 1];
 
vec_ECI = C_b_ECI'*vec_b;

== matlab function GUARD_Toolbox/Physical Subsystems/Aerodynamics/ECI_2_Body ==
  settings: sampleTime=Tsc
  data: vec_ECI input; q input; vec_b output
function  vec_b = ECI_to_body(vec_ECI,q)
%#codegen

% Rotate a vector from the orbital frame to the body frame 
% C_bo = Quaternion rotation matrix
% vec_b = Body frame vector
% vec_ECI = Earth Fixed Inertial frame vector
% q   = Attitude quaternion
q1=q(1);
q2=q(2);
q3=q(3);
q4=q(4);

C_b_ECI = [ -2*q2^2 - 2*q3^2 + 1,  2*q1*q2 + 2*q3*q4,    2*q1*q3 - 2*q2*q4;
          2*q1*q2 - 2*q3*q4,   -2*q1^2 - 2*q3^2 + 1,  2*q1*q4 + 2*q2*q3;
          2*q1*q3 + 2*q2*q4,    2*q2*q3 - 2*q1*q4,   -2*q1^2 - 2*q2^2 + 1];
 
vec_b = C_b_ECI*vec_ECI;

== matlab function GUARD_Toolbox/Physical Subsystems/Atmosphere (PW exp density)/Altitude (oblate spheroid) ==
  data: sys_pos input; alt output
function alt = altitude(sys_pos)
r = norm3(sys_pos); % distance from the center of the Earth
r_n = sys_pos./r; % normalized position vector

% declination and altitude [m] above oblate spheroid
dec = asin(r_n(3));
alt_m = UW.iPlanet.r_E * (r/UW.iPlanet.r_E - (1 - UW.iPlanet.f)/(sqrt(1 - UW.iPlanet.f*(2 - UW.iPlanet.f)*(cos(dec))^2)));

alt = alt_m/1000; % distance from the planet's surface (assuming it's spherical) [Km]

function vec_n = norm3(vec)
vec_n = sqrt(vec(1)^2 + vec(2)^2 + vec(3)^2);

== matlab function GUARD_Toolbox/Physical Subsystems/Equations of Motion (6-DoF Rigid Body, cont)/Rotational Dynamics/compute_q_dot ==
  data: q input; q_dot output; omega input
function q_dot = q_rate(q,omega)
%#codegen

wx=omega(1);
wy=omega(2);
wz=omega(3);

W=[ 0   wz -wy wx;
   -wz  0   wx wy;
    wy -wx  0  wz;
   -wx -wy -wz 0 ];

q_dot=.5*W*q; %unit quaternion rate

== matlab function GUARD_Toolbox/Software Subsystems/UE4 OSC_UDP Interface/OSC_data_convert ==
  data: pos_sim input; pos_OSC output
function  pos_OSC = OSC_data(pos_sim)
%#codegen
n_in=length(pos_sim);
pos_OSC=uint8(zeros(1,(n_in*4)));

pos_OSC=typecast(swapbytes(single(pos_sim)),'uint8');

== matlab function GUARD_Toolbox/Physical Subsystems/Inertia and CoM Evolution/MATLAB Function ==
  data: I_ii input; current_inertia output
function current_inertia = Diag_Matrix(I_ii)
%#codegen

current_inertia = [I_ii(1) 0       0;
                   0       I_ii(1) 0;
                   0       0       I_ii(1)];

== matlab function GUARD_Toolbox/Physical Subsystems/Equations of Motion (6-DoF Rigid Body, cont)/Rotational Dynamics/normalize_quaternion ==
  data: q input; q_n output
function q_n = q_norm(q)
%#codegen

qN=sqrt(q(1)^2 + q(2)^2 + q(3)^2 + q(4)^2);
q_n=q/qN;

== matlab function GUARD_Toolbox/Software Subsystems/UE4 OSC_UDP Interface/OSC_path_generate ==
  data: path_OSC output
function  path_OSC = OSC_obj_path
%#codegen
address='rocket';
path=uint8(address);
% retrives number of input data elements
% n_in=length(path);
front_slash = 47;
four_byte_packet=zeros(1,4);
% format type string
path_to_mod=[front_slash path four_byte_packet];
% adjust length
length_path_to_mod=length(path_to_mod);
final_path_str=path_to_mod(1:length_path_to_mod-mod(length_path_to_mod,4));
% convert to uint8
path_OSC=uint8(final_path_str);

== matlab function GUARD_Toolbox/Software Subsystems/UE4 OSC_UDP Interface/OSC_types_generate ==
  data: pos_sim input; types_OSC output
function  types_OSC = OSC_types(pos_sim)
%#codegen
% retrives number of input data elements
n_in=length(pos_sim);
% generate types string (float = 102)
types=102*ones(1,n_in);
% comma character = 44
comma = 44;
four_byte_packet=zeros(1,4);
% format type string
types_to_mod=[comma types four_byte_packet];
% adjust length
length_types_to_mod=length(types_to_mod);
final_types_str=types_to_mod(1:length_types_to_mod-mod(length_types_to_mod,4));
% convert to uint8
types_OSC=uint8(final_types_str);

== matlab function GUARD_Toolbox/Software Subsystems/UE4 OSC_UDP Interface/coordinates transformation ==
  data: coord_UE4 output; pos_PCI input; Euler_angles input; MV input; vel_PCI input
function  coord_UE4 = coor_trans(pos_PCI, Euler_angles, MV, vel_PCI)
%#codegen
Vn=norm(vel_PCI);
coord_UE4=[100*[pos_PCI(3) pos_PCI(2) pos_PCI(1)] 180/pi*[Euler_angles(3) Euler_angles(2) Euler_angles(1)] MV(4) Vn];
% coord_UE4=[100*[pos_PCI(2) -pos_PCI(3) pos_PCI(1)] 180/pi*[Euler_angles(2) -Euler_angles(3) Euler_angles(1)] MV(4)];

== matlab function GUARD_Toolbox/Physical Subsystems/Fuel Sloshing/Body_2_ECI ==
  settings: sampleTime=Tsc
  data: vec_b input; q input; vec_ECI output
function  vec_ECI = body_to_ECI(vec_b,q)
%#codegen

% Rotate a vector from the orbital frame to the body frame 
% C_bo = Quaternion rotation matrix
% vec_b = Body frame vector
% vec_ECI = Earth Fixed Inertial frame vector
% q   = Attitude quaternion
q1=q(1);
q2=q(2);
q3=q(3);
q4=q(4);

C_b_ECI = [ -2*q2^2 - 2*q3^2 + 1,  2*q1*q2 + 2*q3*q4,    2*q1*q3 - 2*q2*q4;
          2*q1*q2 - 2*q3*q4,   -2*q1^2 - 2*q3^2 + 1,  2*q1*q4 + 2*q2*q3;
          2*q1*q3 + 2*q2*q4,    2*q2*q3 - 2*q1*q4,   -2*q1^2 - 2*q2^2 + 1];
 
vec_ECI = C_b_ECI'*vec_b;

== matlab function GUARD_Toolbox/Physical Subsystems/Gravity Gradient/Gravity Gradient Torque ==
  settings: sampleTime=Tsc
  data: gravity_body input; sys_pos input; ggt output; mu input; current_inertia input
% According to "Spacecraft Attitude Dynamics Hughes 1986", assuming the
% Earth as a perfect rigid sphere with radially simmetric mass 
% distribution, the Gravity Gradient Torque can be computed as
% $3 \frac{mu}{r^3} \cdot g_b \times I g_b$ where $\mu$ is the
% Earth's gravitational constant, r is the distance of the spacecraft from
% the center of the Earth, $g_b$ is the direction of the gravity vector
% expressed in the body frame and $I$ is the inertia matrix.

function  ggt = grav_grad_torque(gravity_body,sys_pos,mu,current_inertia)
%#codegen
%% From Spacecraft Attitude Dynamics Hughes 1986
% 3*mu/r_n^3 * (o3 x I*o3)

g_n = norm3(gravity_body);

o3 = gravity_body/g_n; % Gravity vector direction in body frame

r_n = norm3(sys_pos); % Distance from earth center

grav_field = 3*mu/r_n^3;

ggt = grav_field*crossp(o3, current_inertia*o3);


function vec_n = norm3(vec)
vec_n = sqrt(vec(1)^2 + vec(2)^2 + vec(3)^2);

function w = crossp(u,v)
w=[u(2)*v(3)-u(3)*v(2);
   u(3)*v(1)-u(1)*v(3);
   u(1)*v(2)-u(2)*v(1)];

== matlab function GUARD_Toolbox/Physical Subsystems/Fuel Sloshing/MATLAB Function ==
  data: cons_fuel input; m1 output; alpha_s input; m_fuel_tank input; n_tanks input
function  m1 = sloshing_mass(cons_fuel,alpha_s,m_fuel_tank,n_tanks)
%#codegen

% Fuel tank filling ratio
current_m_fuel_tank = cons_fuel/n_tanks;
tau = current_m_fuel_tank/m_fuel_tank;

lambda = tau*(4*alpha_s-1) + tau^2 * (2 - 4*alpha_s);

m1 = (1 - lambda)*m_Fuel;

== matlab function GUARD_Toolbox/Physical Subsystems/Fuel Sloshing/Sloshing Mass Acceleration/Orbital_2_Body ==
  settings: sampleTime=Tsc
  data: r_o input; q input; r_b output
function  r_b = orbital_to_body(r_o,q)
%#codegen

% Rotate a vector from the orbital frame to the body frame 
% C_bo = Quaternion rotation matrix
% r_b = Body frame vector
% r_o = Orbital frame vector
% q   = Attitude quaternion
q1=q(1);
q2=q(2);
q3=q(3);
q4=q(4);

C_bo = [ -2*q2^2 - 2*q3^2 + 1,  2*q1*q2 + 2*q3*q4,    2*q1*q3 - 2*q2*q4;
          2*q1*q2 - 2*q3*q4,   -2*q1^2 - 2*q3^2 + 1,  2*q1*q4 + 2*q2*q3;
          2*q1*q3 + 2*q2*q4,    2*q2*q3 - 2*q1*q4,   -2*q1^2 - 2*q2^2 + 1];
 
r_b = C_bo*r_o;

== matlab function GUARD_Toolbox/Axes Transformations/Body to ECI ==
  settings: sampleTime=Tsc
  data: vec_b input; q input; vec_ECI output
function  vec_ECI = body_to_ECI(vec_b,q)
%#codegen

% Rotate a vector from the orbital frame to the body frame 
% C_bo = Quaternion rotation matrix
% vec_b = Body frame vector
% vec_ECI = Earth Fixed Inertial frame vector
% q   = Attitude quaternion
q1=q(1);
q2=q(2);
q3=q(3);
q4=q(4);

C_b_ECI = [ -2*q2^2 - 2*q3^2 + 1,  2*q1*q2 + 2*q3*q4,    2*q1*q3 - 2*q2*q4;
          2*q1*q2 - 2*q3*q4,   -2*q1^2 - 2*q3^2 + 1,  2*q1*q4 + 2*q2*q3;
          2*q1*q3 + 2*q2*q4,    2*q2*q3 - 2*q1*q4,   -2*q1^2 - 2*q2^2 + 1];
 
vec_ECI = C_b_ECI'*vec_b;

== matlab function GUARD_Toolbox/Axes Transformations/ECI to Body ==
  settings: sampleTime=Tsc
  data: vec_ECI input; q input; vec_b output
function  vec_b = ECI_to_body(vec_ECI,q)
%#codegen

% Rotate a vector from the orbital frame to the body frame 
% C_bo = Quaternion rotation matrix
% vec_b = Body frame vector
% vec_ECI = Earth Fixed Inertial frame vector
% q   = Attitude quaternion
q1=q(1);
q2=q(2);
q3=q(3);
q4=q(4);

C_b_ECI = [ -2*q2^2 - 2*q3^2 + 1,  2*q1*q2 + 2*q3*q4,    2*q1*q3 - 2*q2*q4;
          2*q1*q2 - 2*q3*q4,   -2*q1^2 - 2*q3^2 + 1,  2*q1*q4 + 2*q2*q3;
          2*q1*q3 + 2*q2*q4,    2*q2*q3 - 2*q1*q4,   -2*q1^2 - 2*q2^2 + 1];
 
vec_b = C_b_ECI*vec_ECI;

== matlab function GUARD_Toolbox/Axes Transformations/From ECEF to ECI ==
  data: t_vec input; vec_ECI output; vec_ECEF input
%% Approximate transformation from ECI coordinates to ECEF
%
% This code does not take in account for small variations in Earth's
% rotation
%
% INPUTS
% t_vec = Time Vector including:
% year % yyyy
% month 
% day  
% hour % 24h
% minute
% second
% 
% vec_ECI = x,y,z [m]
%
% OUTPUTS
% vec_ECEF [m]
%
function vec_ECI = ECEF_to_ECI(t_vec, vec_ECEF)
% Extract time components
year   = t_vec(1);
month  = t_vec(2);
day    = t_vec(3);
hour   = t_vec(4);
minute = t_vec(5);
second = t_vec(6);

vec_ECEF = vec_ECEF(:); % enforce column vector

% Julian Day: count of days since noon March 1 4801 B.C.
% JD = find_Julian(year,month,day,hour,minute,second); 
JD = UW.find_Julian(year,month,day,0,0,0); 
d = JD - 2451545;
T = d/36525;

%% Greenwich Sidereal Time
GST = UW.G_S_T (T, hour, minute, second);

%% Frame Rotation
Rz = [ cos(GST)  sin(GST) 0;
      -sin(GST)  cos(GST) 0;
        0        0        1];
  
vec_ECI = Rz'*vec_ECEF;

== matlab function GUARD_Toolbox/Axes Transformations/From ECEF to LLA ==
  data: vec_ECEF input; LLA output
%% Exact transformation from ECEF coordinates to LLA
%
% Zhu method from : "Conversio of Earth-Centered Earth-Fixed coordinates to
% Geodetic Coordinates." IEEE Transcations on Aerospace and Electronic Systems, 
% Vol.30, No. 3 July 1994.
%
% INPUTS
% t_vec = Time Vector including:
% year % yyyy
% month 
% day  
% hour % 24h
% minute
% second
% 
% vec_ECEF = [X_ECEF; Y_ECEF; Z_ECEF] [m]
%
% OUTPUTS
% LLA [rad; rad; m]
%
function LLA = ECEF_to_LLA(vec_ECEF)

% Extract ECI vector components
X_ECEF = (vec_ECEF(1));
Y_ECEF = (vec_ECEF(2));
Z_ECEF = (vec_ECEF(3));

% Aux variables
% l = iPlanet.e2/2;
r = sqrt(X_ECEF^2 + Y_ECEF^2);
m = (r/UW.iPlanet.r_E)^2;
n = ((1 - UW.iPlanet.e2)*Z_ECEF/UW.iPlanet.r_Ep)^2;
i = -(2*UW.iPlanet.l2 + m + n)/2;
k = UW.iPlanet.l2*(UW.iPlanet.l2 - m - n);
q = (m + n - 4*UW.iPlanet.l2)^3/216 + m*n*UW.iPlanet.l2;
D = sqrt((2*q - m*n*UW.iPlanet.l2)*m*n*UW.iPlanet.l2);
be = i/3 - (q + D)^(1/3) - (q - D)^(1/3);
t = sqrt(sqrt(be^2 - k) - (be + i)/2) - sign(m - n)*sqrt((be - i)/2);
r0 = r/(t + UW.iPlanet.l);
z0 = (1 - UW.iPlanet.e2)*Z_ECEF/(t - UW.iPlanet.l);

lat = atan2(z0, (1 - UW.iPlanet.e2)*r0);
lon = 2*atan2(r - X_ECEF, Y_ECEF) - 2*pi; % Don't subtract 2*pi if there are problems
alt = sign(t - 1 + UW.iPlanet.l)*sqrt((r - r0)^2 + (Z_ECEF - z0)^2);

LLA = [lat;lon;alt];

== matlab function GUARD_Toolbox/Axes Transformations/From ECI to ECEF ==
  data: t_vec input; vec_ECEF output; vec_ECI input
%% Approximate transformation from ECI coordinates to ECEF
%
% This code does not take in account for small variations in Earth's
% rotation
%
% INPUTS
% t_vec = Time Vector including:
% year % yyyy
% month 
% day  
% hour % 24h
% minute
% second
% 
% vec_ECI = x,y,z [m]
%
% OUTPUTS
% vec_ECEF [m]
%
function vec_ECEF = ECI_to_ECEF(t_vec, vec_ECI)
% Extract time components
year   = t_vec(1);
month  = t_vec(2);
day    = t_vec(3);
hour   = t_vec(4);
minute = t_vec(5);
second = t_vec(6);

vec_ECI = vec_ECI(:); % enforce column vector

% Julian Day: count of days since noon March 1 4801 B.C.
% JD = find_Julian(year,month,day,hour,minute,second); 
JD = UW.find_Julian(year,month,day,0,0,0); 
d = JD - 2451545;
T = d/36525;

%% Greenwich Sidereal Time
GST = UW.G_S_T (T, hour, minute, second);

%% Frame rotation
Rz = [ cos(GST)  sin(GST) 0;
      -sin(GST)  cos(GST) 0;
        0        0        1];
  
vec_ECEF = Rz*vec_ECI;

== matlab function GUARD_Toolbox/Axes Transformations/From ECI to LLA ==
  data: t_vec input; LLA output; vec_ECI input
%% Approximate transformation from ECI coordinates to LLA
% where LLA stands for latitude, longitude, and altitude.
%
% This code does not take in account for small variations in Earth's
% rotation
%
% INPUTS
% t_vec = Time Vector including:
% year % yyyy
% month 
% day  
% hour % 24h
% minute
% second
% 
% vec_ECI = x,y,z [m]
%
% OUTPUTS
% lat = latitude [rad]
% lon = latitude [rad]
% alt = latitude [m]
%
function LLA = ECI_to_LLA(t_vec,vec_ECI) 
% Extract time components
year   = t_vec(1);
month  = t_vec(2);
day    = t_vec(3);
hour   = t_vec(4);
minute = t_vec(5);
second = t_vec(6);

% Extract ECI vector components
X_ECI = (vec_ECI(1));
Y_ECI = (vec_ECI(2));
Z_ECI = (vec_ECI(3));

%% Julian Day: count of days since noon March 1 4801 B.C.
% JD = find_Julian(year,month,day,hour,minute,second); 
JD = UW.find_Julian(year,month,day,0,0,0); 
d = JD - 2451545;
T = d/36525;

%% Greenwich Sidereal Time
GST = UW.G_S_T (T, hour, minute, second);

%% LLA
% distance from the center of the Earth
r = sqrt(X_ECI^2 + Y_ECI^2 + Z_ECI^2);

%normalize ECI position
Xn_ECI = X_ECI/r;
Yn_ECI = Y_ECI/r;
Zn_ECI = Z_ECI/r;

% declination, geodetic latitude and altitude above oblate spheroid
dec = asin(Zn_ECI);
lat = atan2(tan(dec),(1 - UW.iPlanet.f)^2);
alt = UW.iPlanet.r_E * (r/UW.iPlanet.r_E - (1 - UW.iPlanet.f)/(sqrt(1 - UW.iPlanet.e2*(cos(dec))^2)));

% right ascension and geocentric longitude of the satellite
ra = atan2(Yn_ECI, Xn_ECI);
lon=atan2(sin(ra - GST), cos(ra - GST));

LLA = [lat;lon;alt];

== matlab function GUARD_Toolbox/Axes Transformations/From LLA to ECEF ==
  data: LLA input; vec_ECEF output
%% Transformation from LLA coordinates to ECEF
%
%
% INPUTS
% LLA:
% lat  = geodetic latitude [rad] (positive North) 
% lon = geodetic longitude [rad] (measured east from the Greenwich meridian)
% alt = altitude [m] (normal to the ellipsod)
% 
%
% OUTPUTS
% vec_ECEF = [X_ECEF;Y_ECEF;Z_ECEF] [m]
%
function vec_ECEF = LLA_to_ECEF(LLA)

lat = LLA(1);
lon = LLA(2);
alt = LLA(3);


R = UW.iPlanet.r_E/sqrt(1 - UW.iPlanet.e2*sin(lat)^2);

R_h = (R + alt);

X_ECEF = R_h*cos(lat)*cos(lon);
Y_ECEF = R_h*cos(lat)*sin(lon);
Z_ECEF = (R_h - UW.iPlanet.e2*R)*sin(lat);

vec_ECEF = [X_ECEF;Y_ECEF;Z_ECEF];

== matlab function GUARD_Toolbox/Axes Transformations/From LVLH to ECI ==
  data: pos_ECI input; vec_ECI output; vel_ECI input; vec_LVLH input
function vec_ECI = LVLH2ECI(pos_ECI,vel_ECI,vec_LVLH)
%#codegen
% This block computes the transformation between the LVLH frame to the ECI 
% frame. The LVLH frame rotates with the orbit and it is always aligned
% such that the X axis is in the local vertical (‘radial’), hence pointing
% outwards, the Z axis is in the direction of the orbit normal, and the 
% Y axis forms a right-handed coordinate system. The origin of the system
% is at the center of mass of the spacecraft. 

% reshape vectors
pos_ECI = pos_ECI(:);
vel_ECI = vel_ECI(:);
vec_LVLH = vec_LVLH(:);

pos_ECI_n = norm3(pos_ECI);
el_R = pos_ECI/pos_ECI_n; % radial unit vector in LVLH frame

pos_vel = crossp(pos_ECI,vel_ECI);
pos_vel_n = norm3(pos_vel);
el_N = pos_vel/pos_vel_n; % normal unit vector in LVLH frame

el_T = crossp(el_N,el_R); % tangential unit vector in LVLH frame

R_ECI_LVLH = [el_R el_T el_N]; % transformation from ECI to LVLH

vec_ECI = R_ECI_LVLH * vec_LVLH;

function vec_n = norm3(vec)
vec_n = sqrt(vec(1)^2 + vec(2)^2 + vec(3)^2);

function w = crossp(u,v)
w=[u(2)*v(3)-u(3)*v(2);
   u(3)*v(1)-u(1)*v(3);
   u(1)*v(2)-u(2)*v(1)];
